simulink model "hw1p3"  (R2021b)
settings: Solver=VariableStepAuto  StartTime=0.0  StopTime=50  RelTol=1e-3
values from neighbouring files (symbols this model uses):
  a = [-(inv_rt+3.*CBs.^0.5) -1.5.*CAs.*CBs.^(-0.5) 0 ... (first row only)    [hw1p3statespacematrix.m]
  b = [inv_rt 0; 0 inv_rt; 0 0]    [hw1p3statespacematrix.m]
  c = [1 0 0; 0 1 0; 0 0 1]    [hw1p3statespacematrix.m]
  CAs = 0.20    (= 0.2)    [hw1p3statespacematrix.m]
  CBs = 0.50    (= 0.5)    [hw1p3statespacematrix.m]
  CCs = 0.75    [hw1p3statespacematrix.m]
  d = [0 0; 0 0; 0 0]    [hw1p3statespacematrix.m]
settings Model: Creator=loren  LastModifiedBy=loren

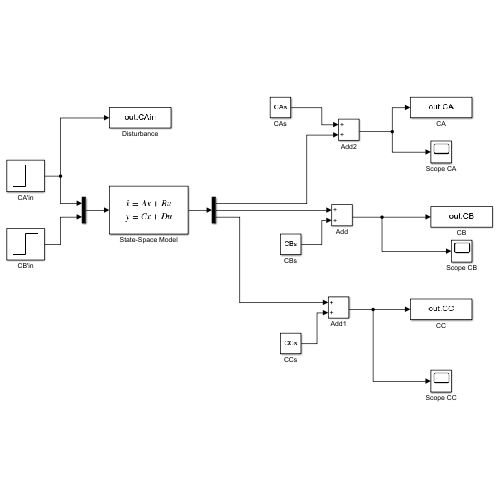
[thumbnail: Simulink's stored preview of the top-level diagram]
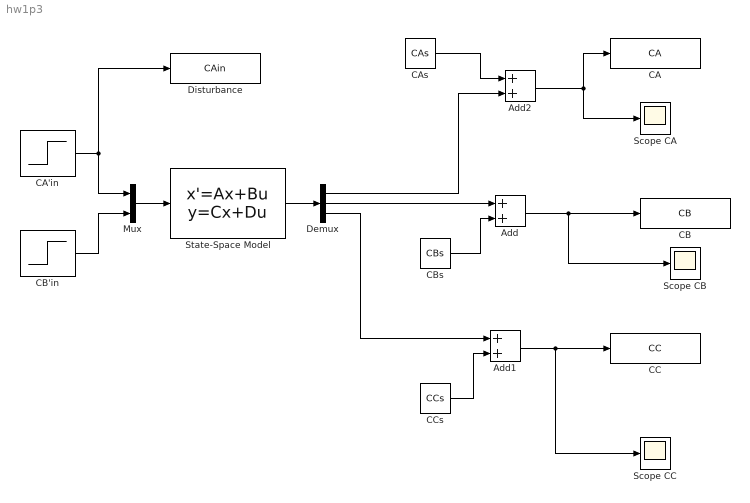
== system hw1p3 ==
  Add : Sum
  Add1 : Sum
  Add2 : Sum
  CA : ToWorkspace  VariableName=CA  SaveFormat=Timeseries  SampleTime=-1
  CA'in : Step  Time=5  After=0.5  SampleTime=0
  CAs : Constant  Value=CAs
  CB : ToWorkspace  VariableName=CB  SaveFormat=Timeseries  SampleTime=-1
  CB'in : Step  Time=0  After=0  SampleTime=0
  CBs : Constant  Value=CBs
  CC : ToWorkspace  VariableName=CC  SaveFormat=Timeseries  SampleTime=-1
  CCs : Constant  Value=CCs
  Demux : Demux  Outputs=3
  Disturbance : ToWorkspace  VariableName=CAin  SaveFormat=Timeseries  SampleTime=-1
  Mux : Mux  Inputs=2
  Scope CA : Scope
  Scope CB : Scope
  Scope CC : Scope
  State-Space Model : StateSpace  A=a  B=b  C=c  D=d  InitialCondition=0
  wires:
  CA'in/1 -> Mux/1, Disturbance/1
  CB'in/1 -> Mux/2
  Mux/1 -> State-Space Model/1
  State-Space Model/1 -> Demux/1
  Demux/2 -> Add/1
  Add/1 -> Scope CB/1, CB/1
  Demux/3 -> Add1/1
  Add1/1 -> Scope CC/1, CC/1
  Add2/1 -> Scope CA/1, CA/1
  Demux/1 -> Add2/2
  CAs/1 -> Add2/1
  CBs/1 -> Add/2
  CCs/1 -> Add1/2
